simulink model "FixedPoint2FixedPoint"  (R2021b)
settings: Solver=VariableStepAuto  StartTime=0.0  StopTime=10.0  RelTol=1e-3
libraries: tiiqmathlib x46
settings Model: Creator=win  LastModifiedBy=win

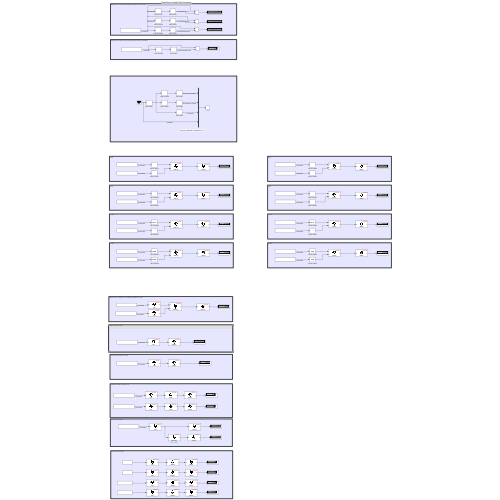
[thumbnail: Simulink's stored preview of the top-level diagram]
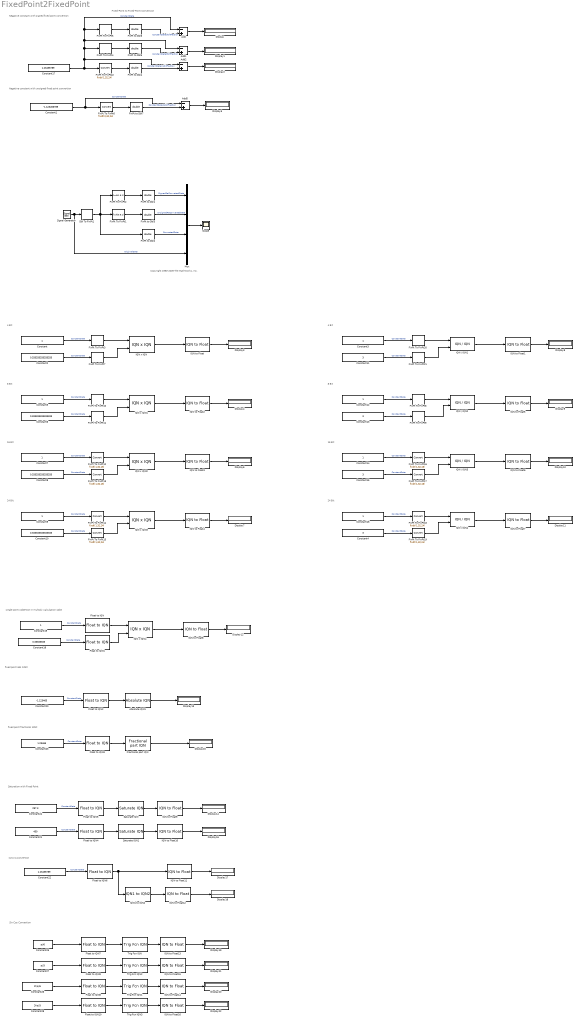
== system FixedPoint2FixedPoint ==
  note: Sin Cos Convertion
  note: Iq to Iq convertion
  note: Saturation with Fixed Point
  note: fixed point fractional 12bit
  note: fixed point abs 12bit
  note: 4 Bit
  note: Negative constant with signed fixed point convertion
  note: Copyright 1990-2009 The MathWorks, Inc.
  note: Fixed-Point to Fixed-Point Conversion
  note: Negative constant with unsigned fixed point convertion
  note: 8 Bit
  note: 16 Bit
  note: 24 Bit
  note: 16 Bit
  note: 4 Bit
  note: 24 Bit
  note: 8 Bit
  note: single point cobertion in multiply calculation 12bit
  Absolute IQN1 : tiiqmathlib/Absolute IQN
      settings: SourceProductBaseCode=TIC2000
  Add{,1..2,5} (4 alike) : Sum  Inputs=-+
  Constant{,3,5,7,9,12,14,16} (8 alike) : Constant
  Constant1 : Constant  Value=-1.123456789
  Constant{2,6,8,10} (4 alike) : Constant  Value=0.333333333333333
  Constant{4,11,13,15} (4 alike) : Constant  Value=3
  Constant17 : Constant  Value=1.23456789
  Constant18 : Constant  Value=0.33333333  OutDataTypeStr=single
  Constant19 : Constant  OutDataTypeStr=single
  Constant20 : Constant  Value=-1.123465  OutDataTypeStr=single
  Constant21 : Constant  Value=450  OutDataTypeStr=single
  Constant22 : Constant  Value=1.23456789  OutDataTypeStr=single
  Constant23 : Constant  Value=1.23465  OutDataTypeStr=single
  Constant24 : Constant  Value=297.3  OutDataTypeStr=single
  Constant25 : Constant  Value=pi/6  OutDataTypeStr=single
  Constant26 : Constant  Value=2*pi/6  OutDataTypeStr=single
  Constant27 : Constant  Value=pi/3  OutDataTypeStr=single
  Constant28 : Constant  Value=2*pi/3  OutDataTypeStr=single
  Dbl To FixPt1 : DataTypeConversion  OutDataTypeStr=fixdt(1,32,2)  RndMeth=Nearest  SaturateOnIntegerOverflow=on
  Display{,1..22} (23 alike) : Display
  FixPt To FixPt1 : DataTypeConversion  OutDataTypeStr=fixdt(0,8,1)  SaturateOnIntegerOverflow=on
  FixPt To FixPt{4,8..11} (5 alike) : DataTypeConversion  OutDataTypeStr=fixdt(1,32,8)  SaturateOnIntegerOverflow=on
  FixPt To FixPt{12..13,16..17} (4 alike) : DataTypeConversion  OutDataTypeStr=fixdt(1,32,16)  SaturateOnIntegerOverflow=on
  FixPt To FixPt{14..15,18..19,22} (5 alike) : DataTypeConversion  OutDataTypeStr=fixdt(1,32,24)  SaturateOnIntegerOverflow=on
  FixPt To FixPt2 : DataTypeConversion  OutDataTypeStr=fixdt(1,8,1)  SaturateOnIntegerOverflow=on
  FixPt To FixPt{3,7,20..21} (4 alike) : DataTypeConversion  OutDataTypeStr=fixdt(1,32,4)  SaturateOnIntegerOverflow=on
  FixPt To FixPt5 : DataTypeConversion  OutDataTypeStr=fixdt(1,32,3)  SaturateOnIntegerOverflow=on
  FixPt To FixPt6 : DataTypeConversion  OutDataTypeStr=fixdt(0,32,24)  SaturateOnIntegerOverflow=on
  FixPt to Dbl{1..7} (7 alike) : DataTypeConversion  OutDataTypeStr=double
  Float to IQN : tiiqmathlib/Float to IQN  Q_value=12
      settings: SourceProductBaseCode=TIC2000
  Float to IQN1 : tiiqmathlib/Float to IQN  Q_value=12
      settings: SourceProductBaseCode=TIC2000
  Float to IQN{6..10} (5 alike) : tiiqmathlib/Float to IQN  Q_value=24
      settings: SourceProductBaseCode=TIC2000
  Float to IQN2 : tiiqmathlib/Float to IQN  Q_value=12
      settings: SourceProductBaseCode=TIC2000
  Float to IQN3 : tiiqmathlib/Float to IQN  Q_value=10
      settings: SourceProductBaseCode=TIC2000
  Float to IQN4 : tiiqmathlib/Float to IQN  Q_value=10
      settings: SourceProductBaseCode=TIC2000
  Float to IQN5 : tiiqmathlib/Float to IQN  Q_value=10
      settings: SourceProductBaseCode=TIC2000
  Fractional part IQN : tiiqmathlib/Fractional part IQN
      settings: SourceProductBaseCode=TIC2000
  IQN / IQN{1..4} (4 alike) : tiiqmathlib/IQN // IQN
      settings: SourceProductBaseCode=TIC2000
  IQN to Float{,1..16} (17 alike) : tiiqmathlib/IQN to Float
      settings: SourceProductBaseCode=TIC2000
  IQN x IQN{,1..3} (4 alike) : tiiqmathlib/IQN x IQN  multiplyOption=Multiply
      settings: SourceProductBaseCode=TIC2000
  IQN x IQN4 : tiiqmathlib/IQN x IQN  multiplyOption=Multiply with rounding and saturation
      settings: SourceProductBaseCode=TIC2000
  IQN1 to IQN2 : tiiqmathlib/IQN1 to IQN2  New_Q=8
      settings: SourceProductBaseCode=TIC2000
  Mux : Mux
  Saturate IQN : tiiqmathlib/Saturate IQN  pos=300  neg=0
      settings: SourceProductBaseCode=TIC2000
  Saturate IQN1 : tiiqmathlib/Saturate IQN  pos=300  neg=0
      settings: SourceProductBaseCode=TIC2000
  Scope : Scope
  Signal Generator : SignalGenerator  WaveForm=sawtooth  Amplitude=5
  Trig Fcn IQN : tiiqmathlib/Trig Fcn IQN  functionOption=_IQsin
      settings: SourceProductBaseCode=TIC2000
  Trig Fcn IQN1 : tiiqmathlib/Trig Fcn IQN  functionOption=_IQsinPU
      settings: SourceProductBaseCode=TIC2000
  Trig Fcn IQN2 : tiiqmathlib/Trig Fcn IQN  functionOption=_IQcos
      settings: SourceProductBaseCode=TIC2000
  Trig Fcn IQN3 : tiiqmathlib/Trig Fcn IQN  functionOption=_IQcosPU
      settings: SourceProductBaseCode=TIC2000
  wires:
  FixPt to Dbl3/1 -> Mux/2  "UnsignedReConvertedData"
  FixPt to Dbl2/1 -> Mux/3  "ConvertedData"
  Dbl To FixPt1/1 -> FixPt To FixPt2/1, FixPt To FixPt1/1, FixPt to Dbl2/1
  FixPt To FixPt1/1 -> FixPt to Dbl3/1
  Mux/1 -> Scope/1
  Signal Generator/1 -> Dbl To FixPt1/1, Mux/4  "OriginalData"
  FixPt To FixPt2/1 -> FixPt to Dbl1/1
  FixPt to Dbl1/1 -> Mux/1  "SignedReConvertedData"
  FixPt To FixPt4/1 -> FixPt to Dbl5/1
  FixPt to Dbl6/1 -> Add/2  "ConstantData3bitFraction"
  FixPt to Dbl5/1 -> Add1/2  "ConstantData8bitFraction"
  FixPt To FixPt5/1 -> FixPt to Dbl6/1
  FixPt to Dbl4/1 -> Add2/2  "ConstantData24bitFraction"
  Constant17/1 -> FixPt To FixPt22/1, Add2/1, Add1/1, Add/1, FixPt To FixPt5/1, FixPt To FixPt4/1  "ConstantData"
  FixPt To FixPt22/1 -> FixPt to Dbl4/1
  Add/1 -> Display/1
  Add1/1 -> Display1/1
  Add2/1 -> Display2/1
  FixPt To FixPt6/1 -> FixPt to Dbl7/1
  Constant1/1 -> Add5/1, FixPt To FixPt6/1  "ConstantData"
  FixPt to Dbl7/1 -> Add5/2  "ConstantData24bitFraction"
  Add5/1 -> Display5/1
  IQN x IQN/1 -> IQN to Float/1
  Constant/1 -> FixPt To FixPt3/1  "ConstantData"
  FixPt To FixPt3/1 -> IQN x IQN/1
  Constant2/1 -> FixPt To FixPt7/1  "ConstantData"
  FixPt To FixPt7/1 -> IQN x IQN/2
  IQN to Float/1 -> Display3/1
  Constant6/1 -> FixPt To FixPt11/1  "ConstantData"
  IQN to Float2/1 -> Display4/1
  FixPt To FixPt10/1 -> IQN x IQN1/1
  IQN x IQN1/1 -> IQN to Float2/1
  Constant5/1 -> FixPt To FixPt10/1  "ConstantData"
  FixPt To FixPt11/1 -> IQN x IQN1/2
  IQN x IQN2/1 -> IQN to Float3/1
  FixPt To FixPt13/1 -> IQN x IQN2/2
  Constant8/1 -> FixPt To FixPt13/1  "ConstantData"
  Constant7/1 -> FixPt To FixPt12/1  "ConstantData"
  FixPt To FixPt12/1 -> IQN x IQN2/1
  IQN to Float3/1 -> Display6/1
  IQN to Float4/1 -> Display7/1
  Constant9/1 -> FixPt To FixPt14/1  "ConstantData"
  IQN x IQN3/1 -> IQN to Float4/1
  FixPt To FixPt14/1 -> IQN x IQN3/1
  FixPt To FixPt15/1 -> IQN x IQN3/2
  Constant10/1 -> FixPt To FixPt15/1  "ConstantData"
  Constant11/1 -> FixPt To FixPt21/1  "ConstantData"
  FixPt To FixPt20/1 -> IQN / IQN1/1
  Constant15/1 -> FixPt To FixPt17/1  "ConstantData"
  IQN to Float6/1 -> Display10/1
  Constant14/1 -> FixPt To FixPt16/1  "ConstantData"
  IQN to Float1/1 -> Display8/1
  IQN / IQN3/1 -> IQN to Float6/1
  FixPt To FixPt19/1 -> IQN / IQN4/2
  Constant4/1 -> FixPt To FixPt19/1  "ConstantData"
  FixPt To FixPt17/1 -> IQN / IQN3/2
  FixPt To FixPt18/1 -> IQN / IQN4/1
  FixPt To FixPt16/1 -> IQN / IQN3/1
  Constant13/1 -> FixPt To FixPt9/1  "ConstantData"
  IQN / IQN2/1 -> IQN to Float5/1
  FixPt To FixPt9/1 -> IQN / IQN2/2
  FixPt To FixPt8/1 -> IQN / IQN2/1
  IQN to Float5/1 -> Display9/1
  IQN / IQN1/1 -> IQN to Float1/1
  FixPt To FixPt21/1 -> IQN / IQN1/2
  Constant3/1 -> FixPt To FixPt20/1  "ConstantData"
  IQN / IQN4/1 -> IQN to Float7/1
  Constant12/1 -> FixPt To FixPt8/1  "ConstantData"
  IQN to Float7/1 -> Display11/1
  Constant16/1 -> FixPt To FixPt18/1  "ConstantData"
  Constant18/1 -> Float to IQN1/1  "ConstantData"
  Float to IQN/1 -> IQN x IQN4/1
  IQN x IQN4/1 -> IQN to Float8/1
  IQN to Float8/1 -> Display12/1
  Constant19/1 -> Float to IQN/1  "ConstantData"
  Float to IQN1/1 -> IQN x IQN4/2
  Absolute IQN1/1 -> Display13/1
  Constant20/1 -> Float to IQN2/1  "ConstantData"
  Float to IQN2/1 -> Absolute IQN1/1
  Fractional part IQN/1 -> Display15/1
  Constant23/1 -> Float to IQN3/1  "ConstantData"
  Float to IQN3/1 -> Fractional part IQN/1
  Float to IQN5/1 -> Saturate IQN/1
  Constant24/1 -> Float to IQN5/1  "ConstantData"
  IQN to Float9/1 -> Display14/1
  Saturate IQN/1 -> IQN to Float9/1
  Constant21/1 -> Float to IQN4/1  "ConstantData"
  Saturate IQN1/1 -> IQN to Float10/1
  Float to IQN4/1 -> Saturate IQN1/1
  IQN to Float10/1 -> Display16/1
  Constant22/1 -> Float to IQN6/1  "ConstantData"
  Float to IQN6/1 -> IQN to Float11/1, IQN1 to IQN2/1
  IQN to Float11/1 -> Display17/1
  IQN1 to IQN2/1 -> IQN to Float12/1
  IQN to Float12/1 -> Display18/1
  Float to IQN7/1 -> Trig Fcn IQN/1
  Float to IQN8/1 -> Trig Fcn IQN1/1
  Float to IQN9/1 -> Trig Fcn IQN2/1
  Float to IQN10/1 -> Trig Fcn IQN3/1
  Constant25/1 -> Float to IQN7/1
  Trig Fcn IQN/1 -> IQN to Float13/1
  Trig Fcn IQN1/1 -> IQN to Float14/1
  Trig Fcn IQN2/1 -> IQN to Float15/1
  Trig Fcn IQN3/1 -> IQN to Float16/1
  IQN to Float13/1 -> Display19/1
  IQN to Float14/1 -> Display20/1
  IQN to Float16/1 -> Display22/1
  IQN to Float15/1 -> Display21/1
  Constant26/1 -> Float to IQN8/1
  Constant27/1 -> Float to IQN9/1
  Constant28/1 -> Float to IQN10/1
